simulink model "LaserBeamStability_v1"  (R2016a)
settings: Solver=FixedStepAuto  StartTime=0.0  StopTime=EndTime  FixedStep=SampleTime  RelTol=1e-3
values from neighbouring files (symbols this model uses):
  A1_IC = pi/4    (= 0.785398163397)    [LaserBeamStability_CommandScript.m]
  A2_IC = pi/4    (= 0.785398163397)    [LaserBeamStability_CommandScript.m]
  A3_IC = pi/4    (= 0.785398163397)    [LaserBeamStability_CommandScript.m]
  A4_IC = pi/4    (= 0.785398163397)    [LaserBeamStability_CommandScript.m]
  ActArm = 3.85    [LaserBeamStability_CommandScript.m]
  b12 = d(14)-d(14)*d(15)/f(2)+d(15)    [LaserBeamStability_CommandScript.m]
  b34 = d(18)-(d(18)*d(19))/f(4)+d(19)    [LaserBeamStability_CommandScript.m]
  c12 = pi/2-2*Beta(2)    [LaserBeamStability_CommandScript.m]
  c34 = pi/2-2*Beta(4)    [LaserBeamStability_CommandScript.m]
  g12 = d(13)-d(13)*d(12)/f(1)+d(12)    [LaserBeamStability_CommandScript.m]
  g34 = d(17)-(d(17)*d(16))/f(3)+d(16)    [LaserBeamStability_CommandScript.m]
  h12 = pi/2-2*Beta(1)    [LaserBeamStability_CommandScript.m]
  h34 = pi/2-2*Beta(3)    [LaserBeamStability_CommandScript.m]
  n_BS = 1.52    [LaserBeamStability_CommandScript.m]
  n_FS = 1.00    (= 1)    [LaserBeamStability_CommandScript.m]
  Noise_Freq = 2*(EndTime)^-1    (= 2)    [LaserBeamStability_CommandScript.m]
  NuetralPoint = (Maximum_Extension-Minimum_Extension)/2    (= 6.25)    [LaserBeamStability_CommandScript.m]
  Optical_Plane_1_Command = [0 0]    [LaserBeamStability_CommandScript.m]
  SampleTime = 1/10    (= 0.1)    [LaserBeamStability_CommandScript.m]
  Sensor12Matx = [a12+b12/d(6) -b12/d(6); g12/d(6) e12-g12/d(6)]    [LaserBeamStability_CommandScript.m]
  Sensor34Matx = [a34+b34/d(10) -b34/d(10); g34/d(10) e34-g34/d(10)]    [LaserBeamStability_CommandScript.m]
  SocketID = TCP_ConnectToServer(IP_ADD, Port, TimeOut)    [LaserBeamStability_CommandScript.m]
  t12 = 2.5    [LaserBeamStability_CommandScript.m]
  t34 = 2.5    [LaserBeamStability_CommandScript.m]
  Target_Command = [0 0]    [LaserBeamStability_CommandScript.m]
undefined symbols (not defined in the file or in its folder): Beta, D, d, f, l, positioner, Td, TLense
(part 2 of 2)

== system LaserBeamStability_v1/GC4/[Rho]/r'o-0001/Beta'-0001 ==
  In1 : Inport
  Add : Sum  Inputs=+-
  Add1 : Sum  Inputs=+++
  Constant : Constant  Value=pi/2
  Constant1 : Constant
  Demux : Demux  Outputs=3
  Divide : Product  Inputs=*/
  Divide1 : Product  Inputs=/*
  Divide2 : Product  Inputs=/*
  Gain : Gain  Gain=-2
  Sum : Sum  Inputs=|++
  Sum1 : Sum  Inputs=++|
  Trigonometric Function : Trigonometry  Operator=tan
  Trigonometric Function1 : Trigonometry  Operator=tan
  Out1 : Outport
  wires:
  In1/1 -> Demux/1
  Demux/1 -> Add1/1
  Constant/1 -> Add1/2
  Demux/2 -> Trigonometric Function/1, Gain/1
  Gain/1 -> Add1/3
  Demux/3 -> Trigonometric Function1/1
  Add1/1 -> Sum1/1, Sum/1
  Sum/1 -> Divide/2
  Constant1/1 -> Add/1, Divide/1
  Trigonometric Function/1 -> Sum1/2
  Trigonometric Function1/1 -> Sum/2
  Sum1/1 -> Divide1/2
  Divide/1 -> Divide2/1, Divide1/1
  Divide1/1 -> Add/2
  Add/1 -> Divide2/2
  Divide2/1 -> Out1/1

== system LaserBeamStability_v1/GC4/[Rho]/r'o-0001/Delta'-0001 ==
  In1 : Inport
  Add1 : Sum  Inputs=++++
  Constant : Constant  Value=pi/2
  Constant1 : Constant
  Demux : Demux  Outputs=3
  Divide : Product  Inputs=*//
  Gain : Gain  Gain=-2
  Trigonometric Function1 : Trigonometry  Operator=tan
  Out1 : Outport
  wires:
  In1/1 -> Demux/1
  Demux/1 -> Add1/1
  Constant/1 -> Add1/2
  Demux/2 -> Gain/1
  Gain/1 -> Add1/3
  Demux/3 -> Trigonometric Function1/1
  Add1/1 -> Divide/2, Divide/3
  Constant1/1 -> Divide/1
  Trigonometric Function1/1 -> Add1/4
  Divide/1 -> Out1/1

== system LaserBeamStability_v1/GC4/[Rho]/r'o-0001/Gamma'-0001 ==
  In2 : Inport
  Add : Sum  Inputs=+-
  Add1 : Sum  Inputs=+++
  Constant : Constant  Value=pi/2
  Constant1 : Constant
  Demux : Demux  Outputs=3
  Divide : Product  Inputs=*/
  Divide1 : Product  Inputs=/*
  Divide2 : Product  Inputs=/*
  Gain : Gain  Gain=-2
  Sum : Sum  Inputs=|++
  Trigonometric Function1 : Trigonometry  Operator=tan
  Out2 : Outport
  wires:
  In2/1 -> Demux/1
  Demux/1 -> Add1/1
  Constant/1 -> Add1/2
  Demux/2 -> Gain/1
  Gain/1 -> Add1/3
  Demux/3 -> Trigonometric Function1/1
  Sum/1 -> Divide/2
  Constant1/1 -> Add/1, Divide/1
  Trigonometric Function1/1 -> Sum/2
  Add1/1 -> Divide1/2, Sum/1
  Divide/1 -> Divide2/1, Divide1/1
  Divide1/1 -> Add/2
  Add/1 -> Divide2/2
  Divide2/1 -> Out2/1

== matlab function LaserBeamStability_v1/PLANT/MATLAB Function1 ==
  data: SocketID input; ErrorReturn output; PositionerID input; AbsolutePosition input
function ErrorReturn = Move_Actuator(SocketID, PositionerID, AbsolutePosition)
%#codegen
%Recieves Absolute Position and which positioner, Reports error codes

[errorCode]=GroupMoveAbsolute(SocketID, PositionerID, AbsolutePosition);


ErrorReturn = errorCode;

== matlab function LaserBeamStability_v1/PLANT/MATLAB Function ==
  data: SocketID input; ErrorReturn output; PositionerID input; AbsolutePosition input
function ErrorReturn = Move_Actuator(SocketID, PositionerID, AbsolutePosition)
%#codegen
%Recieves Absolute Position and which positioner, Reports error codes

[errorCode]=GroupMoveAbsolute(SocketID, PositionerID, AbsolutePosition);


ErrorReturn = errorCode;

== matlab function LaserBeamStability_v1/PLANT/MATLAB Function2 ==
  data: SocketID input; ErrorReturn output; PositionerID input; AbsolutePosition input
function ErrorReturn = Move_Actuator(SocketID, PositionerID, AbsolutePosition)
%#codegen
%Recieves Absolute Position and which positioner, Reports error codes

[errorCode]=GroupMoveAbsolute(SocketID, PositionerID, AbsolutePosition);


ErrorReturn = errorCode;

== matlab function LaserBeamStability_v1/PLANT/MATLAB Function3 ==
  data: SocketID input; ErrorReturn output; PositionerID input; AbsolutePosition input
function ErrorReturn = Move_Actuator(SocketID, PositionerID, AbsolutePosition)
%#codegen
%Recieves Absolute Position and which positioner, Reports error codes

[errorCode]=GroupMoveAbsolute(SocketID, PositionerID, AbsolutePosition);


ErrorReturn = errorCode;
